simulink model "InjCrv_PoI2"  (R2016b)
settings: configuration reference "CodeGenConfigSet" (kept outside this file)
values from neighbouring files (symbols this model uses):
  InjCrv_phiPoI2MaxEOMX_MAP = Calibration.Parameter    [init_InjCrv_PoI2.m]
  InjCrv_phiPoI2MaxEOMX_MAPX = Calibration.Parameter    [init_InjCrv_PoI2.m]
  InjCrv_phiPoI2MaxEOMX_MAPY = Calibration.Parameter    [init_InjCrv_PoI2.m]
  InjCrv_phiPoIMin_C = Calibration.Parameter    [init_InjCrv_PoI2.m]
  InjCrv_stInjCharSetVal_C = Calibration.Parameter    [init_InjCrv_PoI2.m]
libraries: simulink x3, CXLib x2
settings Model: Creator=Administrator  LastModifiedBy=wangrui
settings ConfigSetRef: SourceLocation=Base Workspace

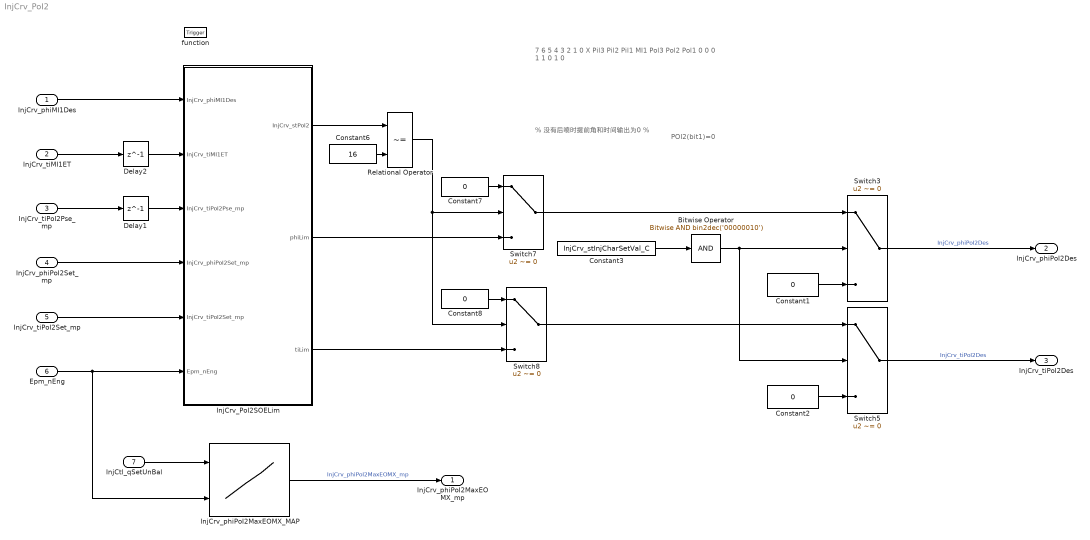
== system InjCrv_PoI2 ==
  note: % 没有后喷时提前角和时间输出为0 %
  note: POI2(bit1)=0
  note: 7
      | 6
      | 5
      | 4
      | 3
      | 2
      | 1
      | 0
      |
      | X
      | Pil3
      | Pil2
      | Pil1
      | MI1
      | Pol3
      | Pol2
      | Pol1
      |
      | 0
      | 0
      | 0
      | 1
      | 1
      | 0
      | 1
      | 0
  InjCrv_phiMI1Des : Inport  Tag=CA  Description=Desired reference angle for the start of MI1  OutMin=-40  OutMax=40  OutDataTypeStr=Angle_CA
  InjCrv_tiMI1ET : Inport  Tag=us  Description=Estimated MI1 energizing time  Port=2  OutMin=-13107  OutMax=13106  OutDataTypeStr=InjTime_us
  InjCrv_tiPoI2Pse_mp : Inport  Tag=us  Description=Minium injection interval between MI1 and PoI2  Port=3  OutMin=-13107  OutMax=13106  OutDataTypeStr=InjTime_us
  InjCrv_phiPoI2Set_mp : Inport  Tag=CA  Description=start of energizing Agngle for PoI2  Port=4  OutMin=-719  OutMax=719  OutDataTypeStr=Angle_CA
  InjCrv_tiPoI2Set_mp : Inport  Tag=us  Description=start of energizing time for PoI2  Port=5  OutMin=-13107  OutMax=13106  OutDataTypeStr=InjTime_us
  Epm_nEng : Inport  Tag=rpm  Description=Engine speed  Port=6  OutMin=0  OutMax=6000  OutDataTypeStr=EngSpeed_rpm
  InjCtl_qSetUnBal : Inport  Tag=mg/hub  Description=Current injection quantity  Port=7  OutMin=-319  OutMax=319  OutDataTypeStr=FuelMass_mg_hub
  function : TriggerPort  TriggerType=function-call  VariantControl=Variant
  Bitwise Operator : simulink/Logic and Bit Operations/Bitwise Operator  logicop=AND  UseBitMask=on  BitMask=bin2dec('00000010')  BitMaskRealWorld=Stored Integer
  Constant{1..2,7..8} (4 alike) : Constant  Value=0  OutDataTypeStr=Inherit: Inherit via back propagation
  Constant3 : Constant  Value=InjCrv_stInjCharSetVal_C
  Constant6 : Constant  Value=16  OutDataTypeStr=uint8
  Delay1 : Delay  DelayLength=1  InitialCondition=0
  Delay2 : Delay  DelayLength=1  InitialCondition=0
  InjCrv_PoI2SOELim : Subsystem
  InjCrv_phiPoI2MaxEOMX_MAP : Lookup_n-D  BreakpointsForDimension1=InjCrv_phiPoI2MaxEOMX_MAPY  BreakpointsForDimension2=InjCrv_phiPoI2MaxEOMX_MAPX  IndexSearchMethod=Linear search  BeginIndexSearchUsingPreviousIndexResult=on  Table=InjCrv_phiPoI2MaxEOMX_MAP  ExtrapMethod=Clip  UseLastTableValue=on  InternalRulePriority=Speed  OutDataTypeStr=Inherit: Inherit via back propagation  SaturateOnIntegerOverflow=on
  Relational Operator : RelationalOperator  Operator=~=  OutDataTypeStr=boolean  RndMeth=Simplest
  Switch3 : Switch  Criteria=u2 ~= 0  InputSameDT=on
  Switch5 : Switch  Criteria=u2 ~= 0  InputSameDT=on
  Switch7 : Switch  Criteria=u2 ~= 0
  Switch8 : Switch  Criteria=u2 ~= 0
  InjCrv_phiPoI2MaxEOMX_mp : Outport  Tag=CA  Description=Maximum PoI2 start of energizing for EOM1-EOM7  OutMin=-719  OutMax=719  OutDataTypeStr=Angle_CA
  InjCrv_phiPoI2Des : Outport  Tag=CA  Description=Desired reference angle for the start of PoI  Port=2  OutMin=-719  OutMax=719  OutDataTypeStr=Angle_CA
  InjCrv_tiPoI2Des : Outport  Tag=us  Description=Desired reference time component for start of PoI2  Port=3  OutMin=-13107  OutMax=13106  OutDataTypeStr=InjTime_us
  wires:
  InjCrv_phiMI1Des/1 -> InjCrv_PoI2SOELim/1(InjCrv_phiMI1Des)
  InjCrv_tiPoI2Pse_mp/1 -> Delay1/1
  InjCrv_PoI2SOELim/2(phiLim) -> Switch7/3
  InjCrv_PoI2SOELim/1(InjCrv_stPoI2) -> Relational Operator/1
  Constant6/1 -> Relational Operator/2
  Relational Operator/1 -> Switch7/2, Switch8/2
  Constant7/1 -> Switch7/1
  Constant8/1 -> Switch8/1
  InjCrv_PoI2SOELim/3(tiLim) -> Switch8/3
  Switch8/1 -> Switch5/1
  InjCrv_phiPoI2Set_mp/1 -> InjCrv_PoI2SOELim/4(InjCrv_phiPoI2Set_mp)
  InjCrv_tiPoI2Set_mp/1 -> InjCrv_PoI2SOELim/5(InjCrv_tiPoI2Set_mp)
  InjCrv_tiMI1ET/1 -> Delay2/1
  Switch5/1 -> InjCrv_tiPoI2Des/1  "InjCrv_tiPoI2Des"
  Switch7/1 -> Switch3/1
  Switch3/1 -> InjCrv_phiPoI2Des/1  "InjCrv_phiPoI2Des"
  Epm_nEng/1 -> InjCrv_PoI2SOELim/6(Epm_nEng), InjCrv_phiPoI2MaxEOMX_MAP/2
  Constant3/1 -> Bitwise Operator/1
  Constant2/1 -> Switch5/3
  Bitwise Operator/1 -> Switch3/2, Switch5/2
  Constant1/1 -> Switch3/3
  InjCtl_qSetUnBal/1 -> InjCrv_phiPoI2MaxEOMX_MAP/1
  InjCrv_phiPoI2MaxEOMX_MAP/1 -> InjCrv_phiPoI2MaxEOMX_mp/1  "InjCrv_phiPoI2MaxEOMX_mp"
  Delay2/1 -> InjCrv_PoI2SOELim/2(InjCrv_tiMI1ET)
  Delay1/1 -> InjCrv_PoI2SOELim/3(InjCrv_tiPoI2Pse_mp)

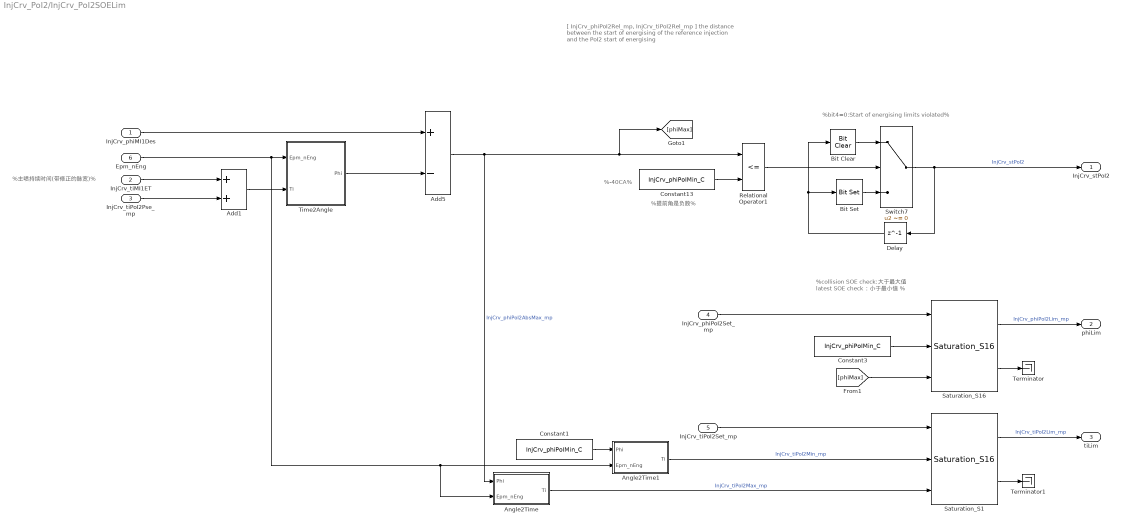
== system InjCrv_PoI2/InjCrv_PoI2SOELim ==
  note: %-40CA%
  note: %bit4=0:Start of energising limits violated%
  note: [ InjCrv_phiPoI2Rel_mp, InjCrv_tiPoI2Rel_mp ]
      | the distance between the start of energising of
      | the reference injection and the PoI2 start of energising
  note: %提前角是负数%
  note: %collision SOE check:大于最大值
      | latest SOE check：小于最小值 %
  note: %主喷持续时间(带修正的脉宽)%
  InjCrv_phiMI1Des : Inport
  InjCrv_tiMI1ET : Inport  Port=2
  InjCrv_tiPoI2Pse_mp : Inport  Port=3
  InjCrv_phiPoI2Set_mp : Inport  Port=4
  InjCrv_tiPoI2Set_mp : Inport  Port=5
  Epm_nEng : Inport  Port=6
  Add1 : Sum  OutDataTypeStr=Inherit: Inherit via back propagation  SaturateOnIntegerOverflow=on  InputSameDT=on
  Add5 : Sum  Inputs=+-  SaturateOnIntegerOverflow=on  InputSameDT=on
  Angle2Time : Subsystem
  Angle2Time1 : Subsystem
  Bit Clear : simulink/Logic and Bit Operations/Bit Clear  iBit=4
  Bit Set : simulink/Logic and Bit Operations/Bit Set  iBit=4
  Constant1 : Constant  Value=InjCrv_phiPoIMin_C
  Constant13 : Constant  Value=InjCrv_phiPoIMin_C
  Constant3 : Constant  Value=InjCrv_phiPoIMin_C
  Delay : Delay  DelayLength=1  InitialCondition=0
  Relational Operator1 : RelationalOperator  Operator=<=  OutDataTypeStr=boolean  RndMeth=Simplest  InputSameDT=on
  Saturation_S1 : CXLib/Saturation_S16
  Saturation_S16 : CXLib/Saturation_S16
  Switch7 : Switch  Criteria=u2 ~= 0
  Terminator : Terminator
  Terminator1 : Terminator
  Time2Angle : Subsystem
  InjCrv_stPoI2 : Outport
  phiLim : Outport  Port=2
  tiLim : Outport  Port=3
  wires:
  Epm_nEng/1 -> Angle2Time/2(Epm_nEng), Angle2Time1/2(Epm_nEng), Time2Angle/1(Epm_nEng)
  Add5/1 -> Angle2Time/1(Phi), Relational Operator1/1, [phiMax]  "InjCrv_phiPoI2AbsMax_mp"
  Constant13/1 -> Relational Operator1/2
  InjCrv_phiPoI2Set_mp/1 -> Saturation_S16/1
  Constant3/1 -> Saturation_S16/2
  Relational Operator1/1 -> Switch7/2
  Switch7/1 -> Delay/1, InjCrv_stPoI2/1  "InjCrv_stPoI2"
  Delay/1 -> Bit Clear/1, Bit Set/1
  Saturation_S16/1 -> phiLim/1  "InjCrv_phiPoI2Lim_mp"
  InjCrv_phiMI1Des/1 -> Add5/1
  InjCrv_tiPoI2Set_mp/1 -> Saturation_S1/1
  Angle2Time/1(Ti) -> Saturation_S1/3  "InjCrv_tiPoI2Max_mp"
  InjCrv_tiPoI2Pse_mp/1 -> Add1/2
  InjCrv_tiMI1ET/1 -> Add1/1
  Add1/1 -> Time2Angle/2(Ti)
  Time2Angle/1(Phi) -> Add5/2
  [phiMax] -> Saturation_S16/3
  Saturation_S16/2 -> Terminator/1
  Saturation_S1/2 -> Terminator1/1
  Saturation_S1/1 -> tiLim/1  "InjCrv_tiPoI2Lim_mp"
  Constant1/1 -> Angle2Time1/1(Phi)
  Angle2Time1/1(Ti) -> Saturation_S1/2  "InjCrv_tiPoI2Min_mp"
  Bit Set/1 -> Switch7/3
  Bit Clear/1 -> Switch7/1

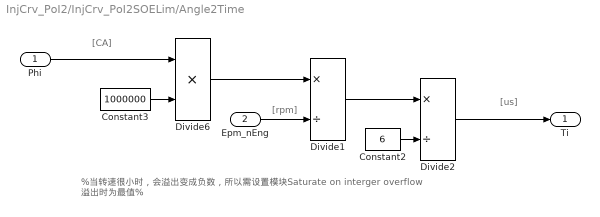
== system InjCrv_PoI2/InjCrv_PoI2SOELim/Angle2Time ==
  note: %当转速很小时，会溢出变成负数，所以需设置模块Saturate on interger overflow
      | 溢出时为最值%
  note: [us]
  note: [rpm]
  note: [CA]
  Phi : Inport
  Epm_nEng : Inport  Port=2
  Constant2 : Constant  Value=6  VectorParams1D=off  OutDataTypeStr=uint8
  Constant3 : Constant  Value=1000000  VectorParams1D=off  OutDataTypeStr=uint32
  Divide1 : Product  Inputs=*/  OutDataTypeStr=fixdt(1,32,3)  SaturateOnIntegerOverflow=on
  Divide2 : Product  Inputs=*/  OutDataTypeStr=Inherit: Inherit via back propagation  SaturateOnIntegerOverflow=on
  Divide6 : Product  Inputs=**  OutDataTypeStr=fixdt(1,32,3)  SaturateOnIntegerOverflow=on
  Ti : Outport
  wires:
  Divide2/1 -> Ti/1
  Epm_nEng/1 -> Divide1/2
  Phi/1 -> Divide6/1
  Divide6/1 -> Divide1/1
  Constant2/1 -> Divide2/2
  Divide1/1 -> Divide2/1
  Constant3/1 -> Divide6/2

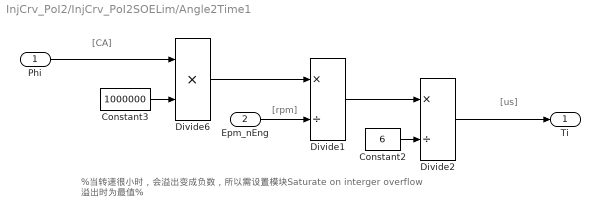
== system InjCrv_PoI2/InjCrv_PoI2SOELim/Angle2Time1 ==
  note: [CA]
  note: [rpm]
  note: [us]
  note: %当转速很小时，会溢出变成负数，所以需设置模块Saturate on interger overflow
      | 溢出时为最值%
  Phi : Inport
  Epm_nEng : Inport  Port=2
  Constant2 : Constant  Value=6  VectorParams1D=off  OutDataTypeStr=uint8
  Constant3 : Constant  Value=1000000  VectorParams1D=off  OutDataTypeStr=uint32
  Divide1 : Product  Inputs=*/  OutDataTypeStr=fixdt(1,32,3)  SaturateOnIntegerOverflow=on
  Divide2 : Product  Inputs=*/  OutDataTypeStr=Inherit: Inherit via back propagation  SaturateOnIntegerOverflow=on
  Divide6 : Product  Inputs=**  OutDataTypeStr=fixdt(1,32,3)  SaturateOnIntegerOverflow=on
  Ti : Outport
  wires:
  Constant3/1 -> Divide6/2
  Divide1/1 -> Divide2/1
  Constant2/1 -> Divide2/2
  Divide6/1 -> Divide1/1
  Phi/1 -> Divide6/1
  Epm_nEng/1 -> Divide1/2
  Divide2/1 -> Ti/1

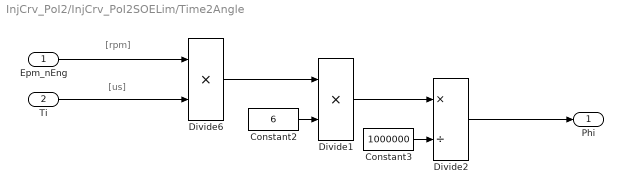
== system InjCrv_PoI2/InjCrv_PoI2SOELim/Time2Angle ==
  note: [us]
  note: [rpm]
  Epm_nEng : Inport
  Ti : Inport  Port=2
  Constant2 : Constant  Value=6  VectorParams1D=off  OutDataTypeStr=uint8
  Constant3 : Constant  Value=1000000  VectorParams1D=off  OutDataTypeStr=uint32
  Divide1 : Product  Inputs=**  OutDataTypeStr=fixdt(1,32,3)  SaturateOnIntegerOverflow=on
  Divide2 : Product  Inputs=*/  OutDataTypeStr=Inherit: Inherit via back propagation  SaturateOnIntegerOverflow=on
  Divide6 : Product  Inputs=**  OutDataTypeStr=fixdt(1,32,3)  SaturateOnIntegerOverflow=on
  Phi : Outport
  wires:
  Epm_nEng/1 -> Divide6/1
  Ti/1 -> Divide6/2
  Divide6/1 -> Divide1/1
  Constant2/1 -> Divide1/2
  Divide1/1 -> Divide2/1
  Constant3/1 -> Divide2/2
  Divide2/1 -> Phi/1
